simulink model "TestPythonIntegrationModel"  (R2023a)
settings: Solver=VariableStepAuto  StartTime=0.0  StopTime=10.0  RelTol=1e-3
settings Model: Creator=zacha  LastModifiedBy=zacha

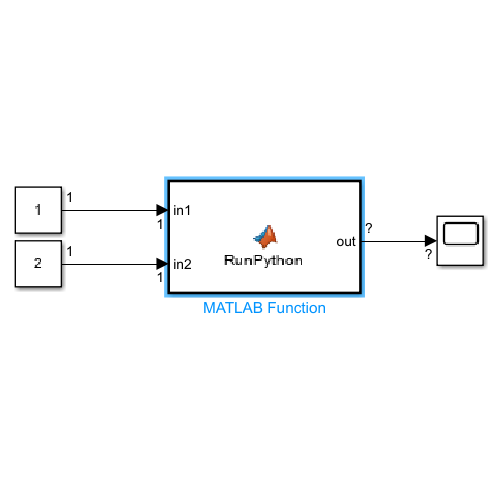
[thumbnail: Simulink's stored preview of the top-level diagram]
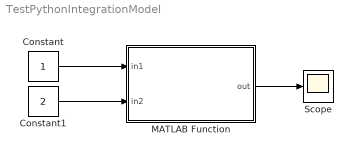
== system TestPythonIntegrationModel ==
  Constant : Constant
  Constant1 : Constant  Value=2
  MATLAB Function : MATLAB Function  TreatAsAtomicUnit=on
  Scope : Scope
  wires:
  Constant/1 -> MATLAB Function/1(in1)
  Constant1/1 -> MATLAB Function/2(in2)
  MATLAB Function/1(out) -> Scope/1

== matlab function TestPythonIntegrationModel/MATLAB Function ==
  data: in1 input; out output; in2 input
function out = RunPython(in1, in2)
    out = 0; % Has to be preassigned, otherwise Simulink throws an error
    coder.extrinsic('Scripts/py.Example.test') % Python functions have to be run extrinsically, meaning no C code generated
    out = py.Example.test(in1,in2);
end
